simulink model "openLoop"  (R2025b)
settings: Solver=FixedStepAuto  StartTime=0.0  StopTime=inf  FixedStep=0.01  RelTol=1e-3
model workspace (MAT data in the model file):
  freq = 0.87
settings Model: Creator=marko  LastModifiedBy=Marko
settings DebuggingCC: UnconnectedInputMsg=warning  UnconnectedOutputMsg=warning  UnconnectedLineMsg=warning
settings ModelReferenceCC: EnableRefExpFcnMdlSchedulingChecks=on
settings RTWCC: GPUComputeCapability=3.5  DLArmComputeVersion=19.05

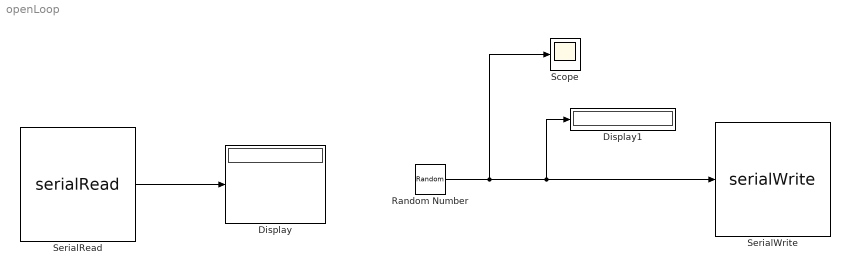
== system openLoop ==
  Display : Display
  Display1 : Display
  Random Number : RandomNumber  SampleTime=0.1
  Scope : Scope
      settings: ActiveDisplayYMinimum=-2.8992700534479647  ActiveDisplayYMaximum=2.3188875433773495
  SerialRead : M-S-Function  FunctionName=serialRead  Parameters='COM4'
  SerialWrite : M-S-Function  FunctionName=serialWrite  Parameters='COM4'
  wires:
  SerialRead/1 -> Display/1
  Random Number/1 -> Scope/1, Display1/1, SerialWrite/1
